simulink model "SimulatorModel"  (Simulink 10.1)
settings: Solver=ode8  StartTime=0.0  StopTime=100000  FixedStep=time_step  RelTol=1e-3
StartFcn:
  | copyfile(char(CurrentFolder + "\3DModels\" + string(MODELO_3D)), char(CurrentFolder + "\" + string(MODELO_3D)));
StopFcn:
  | delete(MODELO_3D)
values from neighbouring files (symbols this model uses):
  Aileron_Trim = 0    [InitialState.m]
  Elevator_Trim = 0    [InitialState.m]    (also in main.m)
  Engine_Trim = 0    [InitialState.m]    (also in main.m)
  GeoDate_Ap = GeoDate_ApIndex(randi([1,length(GeoDate_ApIndex)],1))    [main.m]
  GeoDate_Day = datenum(char(today("datetime")),'dd-mmm-yyyy')-datenum(char("01-January-" + GeoDate_Clock(1)'),'dd-mmm-yyyy')    [main.m]
  GeoDate_LatLongElv = [dms2degrees(Lat) dms2degrees(Long) Elv]    [main.m]
  GeoDate_Time = GeoDate_Clock(4) * 3600 + GeoDate_Clock(5) * 60 + GeoDate_Clock(6)    [main.m]
  Mission = 0    [main.m]
  Mission_Data = [0,0,0,0,0;0,0,0,0,0;0,0,0,0,0]    [main.m]
  p_ini = 0    [InitialState.m]
  phi_ini = 0*pi/180    (= 0)    [InitialState.m]    (also in main.m)
  psi_ini = 0*pi/180    (= 0)    [InitialState.m]    (also in main.m = -1.1815879036)
  q_ini = 0    [InitialState.m]
  r_ini = 0    [InitialState.m]
  Rudder_Trim = 0    [InitialState.m]
  theta_ini = 1*pi/180    (= 0.0174532925199)    [InitialState.m]    (also in main.m = 0)
  time_step = 0.200    (= 0.2)    [main.m]
  u_ini = 0    [InitialState.m]    (also in main.m)
  v_ini = 0    [InitialState.m]    (also in main.m)
  w_ini = 0    [InitialState.m]    (also in main.m)
  x_ini = 0    [InitialState.m]    (also in main.m)
  y_ini = 0    [InitialState.m]    (also in main.m)
  z_ini = h    (= 7350)    [InitialState.m]    (also in main.m = 0)
undefined symbols (not defined in the file or in its folder): AoA_alpha_max, AoA_beta_max, b, c, cargo_mass, CD0_interp, CD_ajus_coef, CD_beta_interp, CD_mach_reg, CDde, CDflap, CDgear, CDi, CDsb, CDsp, CL_ajus_coef, CL_alpha_interp, CL_alpha_reg, Clb, Clda_interp, CLde, Cldr, Clp, Clr, Cm0, Cm_alpha, Cmadot, Cmde_ajus_coef, Cmde_interp, Cmq, Cnb, Cndr, Cnr, Coef_Aileron_Beta, Coef_Aileron_Phi, Coef_Aileron_Rudder, Coef_Elevator_Alpha, Coef_Rudder_Aileron, Coef_Rudder_Beta, CYb, dCLflap, dfuel, dfuel0, e0_0, e1_0, e2_0, e3_0, fuel, fuel_density, fuel_max, g, Ixx, Ixz, Iyy, Izz, kCDge_interp, kCLge_interp, kCLsb, kCLsp, KT ... (+20)
libraries: aerolibconvert2 x17, aerolibutil x14, dsppolyfun x7, aerolibactuator x5, sharedtransform x4, robotcorelib x4, simulink x3, aerolibanim x3, visionstatistics x3, vrlib x2, dspsnks4 x1, dspvision x1
(part 1 of 3)
settings Model: Creator=AngelDanielVR_2022  LastModifiedBy=eldan  EnablePacing=on
settings Model: SuppressorTable=|
  | <?xml version="1.0" encoding="UTF-8" standalone="yes" ?>
  | <!DOCTYPE boost_serialization>
  | <boost_serialization signature="serialization::archive" version="17">
  | <DiagnosticSuppressor class_id="0" tracking_level="0" version="6">
  | 	<Table class_id="1" tracking_level="0" version="0">
  | 		<count>1</count>
  | 		<bucket_count>8</bucket_count>
  | 		<item_version>0</item_version>
  | 		<item class_id="2" tracking_level="0" version="0">
  | 			<first class_id="3" tracking_level="0" version="6">
  | 				<Source class_id="4" tracking_level="0" version="0">
  | 					<count>1</count>
  | 					<item_version>0</item_version>
  | 					<item>SimulatorModel/Fuerzas Aerodinamicas/Divide</item>
  | 				</Source>
  | 			</first>
  | 			<second class_id="5" tracking_level="0" version="6">
  | 				<SuppressedData class_id="6" tracking_level="0" version="0">
  | 					<count>1</count>
  | 					<bucket_count>8</bucket_count>
  | 					<item_version>0</item_version>
  | 					<item class_id="7" tracking_level="0" version="0">
  | 						<first class_id="8" tracking_level="0" version="6">
  | 							<ID>Simulink:blocks:DivideByZero</ID>
  | 							<Cause>
  | 								<Source>
  | 									<count>0</count>
  | 									<item_version>0</item_version>
  | 								</Source>
  | 							</Cause>
  | 						</first>
  | 						<second class_id="9" tracking_level="0" version="6">
  | 							<Comment></Comment>
  | 							<User>eldan</User>
  | 							<LastModified class_id="10" tracking_level="0" version="0">
  | 								<ptime_date class_id="11" tracking_level="0" version="0">
  | 									<date>20220312</date>
  | 								</ptime_date>
  | 								<ptime_time_duration class_id="12" tracking_level="0" version="1">
  | 									<is_special>0</is_special>
  | 									<time_duration_hours>20</time_duration_hours>
  | 									<time_duration_minutes>16</time_duration_minutes>
  | 									<time_duration_seconds>47</time_duration_seconds>
  | 									<time_duration_fractional_seconds>0</time_duration_fractional_seconds>
  | 								</ptime_time_duration>
  | 							</LastModified>
  | 							<SuppressionType>0</SuppressionType>
  | 						</second>
  | 					</item>
  | 				</SuppressedData>
  | 			</second>
  | 		</item>
  | 	</Table>
  | </DiagnosticSuppressor>
  | 
  | </boost_serialization>
  | 
  | </boost_serialization>
settings DataIOCC: SaveFormat=Dataset  ReturnWorkspaceOutputs=on  ReturnWorkspaceOutputsName=Simulation
settings OptimizationCC: LifeSpan=auto
settings DebuggingCC: UnderspecifiedInitializationDetection=Simplified  MergeDetectMultiDrivingBlocksExec=error  SFUnexpectedBacktrackingDiag=error  SFNoUnconditionalDefaultTransitionDiag=error  SFExecutionAtInitializationDiag=warning  ArithmeticOperatorsInVariantConditions=error
settings HardwareCC: ProdBitPerPointer=64  ProdBitPerSizeT=64  ProdBitPerPtrDiffT=64  ProdLargestAtomicFloat=Float  ProdIntDivRoundTo=Zero  ProdEndianess=LittleEndian  ProdWordSize=64  ProdHWDeviceType=Intel->x86-64 (Windows64)
settings ModelReferenceCC: PropagateSignalLabelsOutOfModel=on
settings SFSimCC: SimUseLocalCustomCode=on  CustomCodeUndefinedFunction=FilterOut
settings RTWCC: RTWUseLocalCustomCode=on
settings CodeAppCC: StateflowObjectComments=off
settings GRTTargetCC: TargetLangStandard=C99 (ISO)  CombineOutputUpdateFcns=on  GRTInterface=off
settings ConfigComp: CovMetricSettings=dwe  CovHtmlReporting=off  CovSaveCumulativeToWorkspaceVar=off  CovSaveSingleToWorkspaceVar=off  CovExternalEMLEnable=on

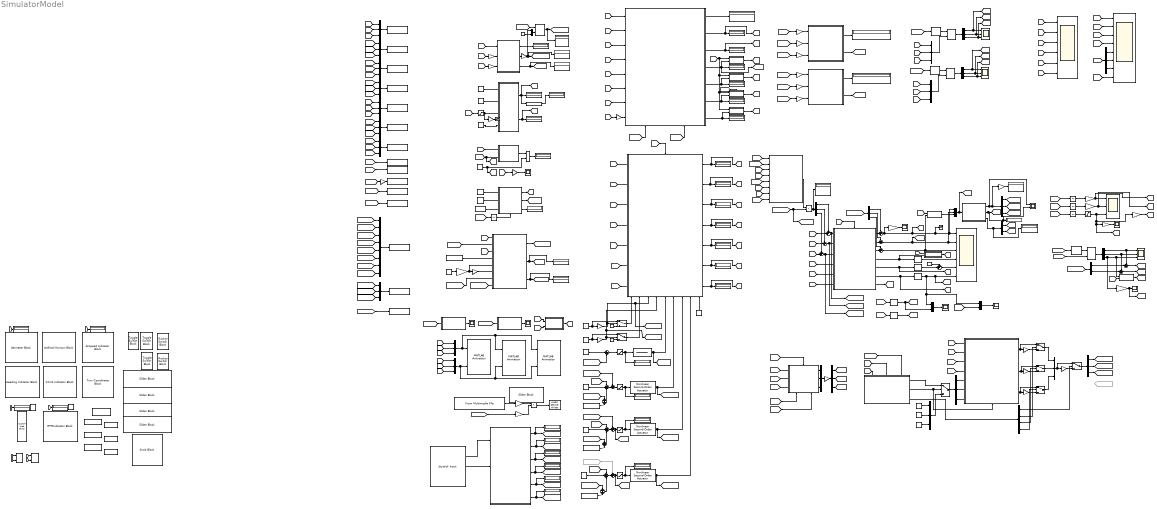
== system SimulatorModel ==
  note: Engine %
  note: Fuel %
  note: Auto-Pilot
  note: ft
  note: ALT
  note: knots
  note: VEL
  note: deg
  note: HDG
  note: Wind Control
  note: Flight Assistance
  note: Gear
  note: Speedbrakes
  note: Spoilers
  "       " : Constant  Value=mass0
  "          " : Constant  Value=fuel
  "               " : Constant  Value=cargo_mass
  6DOF (Ejes Cuerpo) : Subsystem
      settings: PortSchema="{\"entries\":[{\"content\":{\"sides\":[{\"content\":{\"connectorIds\":[\"In1\",\"In2\",\"In3\",\"In4\",\"In5\",\"In6\"]},\"type\":\"ConnectorPlacement.EquallySpacedRectSide\",\"uuid\":\"e513d8e1-8e1d-4192-a11f-b667e9f47cd4\"},{\"content\":{\"connectorIds\":[\"Out1\",\"Out2\",\"Out3\",\"Out4\",\"Out5\",\"Out6\",\"Out7\"],\"side\":\"RIGHT\"},\"type\":\"ConnectorPlacement.EquallySpacedRectSide\",\"uuid\":\"fc5bffb2-c734-419d-b044-938a48a874f8\"},{\"content\":{\"connectorIds\":[\"In7\"],\"side\":\"TOP\"},\"type\":\"ConnectorPlacement.EquallySpacedRectSide\",\"uuid\":\"e4739993-ca2d-4725-a873-646bc3002720\"}]},\"type\":\"ConnectorPlacement.EquallySpacedConnector\",\"uuid\":\"4b4d31a3-c546-405e-8f8c-e6c94c8ecc35\"}],\"packageUris\":[\"http://schema.mathworks.com/mf0/Connector/19700101\"],\"version\":\"1.0\"}"
  ALT : Gain
  Abs : Abs
  Aileron Position : Constant  Value=0
  Airspeed Indicator1 : AirspeedIndicatorBlock  LabelPosition=Hide  ScaleMin=60  ScaleMax=717  ScaleColors=DataTag1
  Altimeter : AltimeterBlock  LabelPosition=Hide
  Altitude Navigation : simulink/Sinks/XY Graph  xmin=0  xmax=500  ymin=0  ymax=8000  st=1
  Altura Autopiloto : Constant  Value=24114
  Angle Conversion{,1..2,6..7} (5 alike) : aerolibconvert2/Angle Conversion  IU=rad  OU=deg
  Animacion Aeronave 3D Back : aerolibanim/MATLAB Animation  Tag=Matlab Animation 6 DOF  Vehicles=1  Geometries=MODELO_3D  BoundingBoxCoordinates=MODELO_3D_Data_Box  CameraOffset=MODELO_3D_DataBack_Offset  CameraViewAngle=2  SampleTime=time_step  FigurePosition=[37,8.020000e+01,396,3.184000e+02]
      settings: SourceProductBaseCode=AE
  Animacion Aeronave 3D ISO : aerolibanim/MATLAB Animation  Tag=Matlab Animation 6 DOF  Vehicles=1  Geometries=MODELO_3D  BoundingBoxCoordinates=MODELO_3D_Data_Box  CameraOffset=MODELO_3D_DataISO_Offset  CameraViewAngle=2  SampleTime=time_step  FigurePosition=[1.018000e+02,4.602000e+02,4.008000e+02,3.080000e+02]
      settings: SourceProductBaseCode=AE
  Animacion Aeronave 3D Side : aerolibanim/MATLAB Animation  Tag=Matlab Animation 6 DOF  Vehicles=1  Geometries=MODELO_3D  BoundingBoxCoordinates=MODELO_3D_Data_Box  CameraOffset=MODELO_3D_DataSide_Offset  CameraViewAngle=2  SampleTime=time_step  FigurePosition=[7.138000e+02,1.226000e+02,7.064000e+02,4.224000e+02]
      settings: SourceProductBaseCode=AE
  Artificial Horizon : ArtificialHorizonBlock  LabelPosition=Hide
  Asistencia en Vuelo : Subsystem
      settings: PortSchema="{\"entries\":[{\"content\":{\"sides\":[{\"content\":{\"connectorIds\":[\"In1\",\"In2\",\"In3\"]},\"type\":\"ConnectorPlacement.EquallySpacedRectSide\",\"uuid\":\"2b982a28-1fea-4abf-9de3-2f9de9411225\"},{\"content\":{\"connectorIds\":[\"Out1\",\"Out2\",\"Out3\"],\"side\":\"RIGHT\"},\"type\":\"ConnectorPlacement.EquallySpacedRectSide\",\"uuid\":\"2f2ccd38-6861-4845-9efc-cf53ec30643e\"},{\"content\":{\"connectorIds\":[\"In4\"],\"side\":\"TOP\"},\"type\":\"ConnectorPlacement.EquallySpacedRectSide\",\"uuid\":\"10eced36-af19-42c5-8d6d-546cf7986fc2\"},{\"content\":{\"connectorIds\":[\"In5\",\"In6\"],\"side\":\"BOTTOM\"},\"type\":\"ConnectorPlacement.EquallySpacedRectSide\",\"uuid\":\"486c9866-702d-4628-bb5b-4c00364c2671\"}]},\"type\":\"ConnectorPlacement.EquallySpacedConnector\",\"uuid\":\"8a4f78da-55c7-44fd-bc59-53ea1e78315a\"}],\"packageUris\":[\"http://schema.mathworks.com/mf0/Connector/19700101\"],\"version\":\"1.0\"}"
  Audio Device Writer : dspsnks4/Audio Device Writer  Driver=DirectSound  Device=Default  InheritSampleRate=on  SampleRate=44100  BitDepth=16-bit integer  BufferSize=4096  NumBuffers=10  DefaultOutputChannelMapping=on  OutputChannelMapping=1:2  OutputNumUnderrunSamples=off  DriverIdx=1  DeviceWarnFlag=''
  Auto-Piloto : Subsystem
      settings: PortSchema="{\"entries\":[{\"content\":{\"sides\":[{\"content\":{\"connectorIds\":[\"In1\",\"In2\",\"In3\",\"In4\",\"In5\",\"In6\",\"In7\"]},\"type\":\"ConnectorPlacement.EquallySpacedRectSide\",\"uuid\":\"540fb58f-a9c8-4ad4-9356-3d566afe9f2d\"},{\"content\":{\"connectorIds\":[\"Out1\",\"Out2\",\"Out3\"],\"side\":\"RIGHT\"},\"type\":\"ConnectorPlacement.EquallySpacedRectSide\",\"uuid\":\"002c5e45-ef8b-4bc5-a5df-6a486272560c\"},{\"content\":{\"connectorIds\":[],\"side\":\"TOP\"},\"type\":\"ConnectorPlacement.EquallySpacedRectSide\",\"uuid\":\"228a911a-da3e-4d63-8be4-0617bff602d3\"},{\"content\":{\"connectorIds\":[\"In8\"],\"side\":\"BOTTOM\"},\"type\":\"ConnectorPlacement.EquallySpacedRectSide\",\"uuid\":\"7f0ae31e-3482-443b-902a-85f32887179f\"}]},\"type\":\"ConnectorPlacement.EquallySpacedConnector\",\"uuid\":\"3a82b01a-db7e-44ad-a37b-33b4a4c7be3f\"}],\"packageUris\":[\"http://schema.mathworks.com/mf0/Connector/19700101\"],\"version\":\"1.0\"}"
  Brake Force System : Subsystem
  Climb Rate Indicator : ClimbIndicatorBlock  LabelPosition=Hide  ScaleMax=20000
  Constant : Constant  Value=Aileron_Trim
  Constant1 : Constant  Value=Rudder_Trim
  Constant2 : Constant  Value=Elevator_Trim
  Constant3 : Constant  Value=Engine_Trim
  Constant4 : Constant
  Constant5 : Constant
  Constant6 : Constant  Value=0
  Constant7 : Constant  Value=90
  Control ON/OFF Asistencia en Vuelo : Gain
  Demux{,1..3,5..8,10..11} (10 alike) : Demux  Outputs=3
  Demux12 : Demux
  Demux4 : Demux  Outputs=2
  Demux9 : Demux  Outputs=2
  Densidad : Display
  Densidad a  Nivel del Mar : Constant  Value=rho0
  Dirección Autopiloto : Constant  Value=22
  Display{,1..12} (13 alike) : Display
  Edit : EditField  LabelPosition=Hide  ShowInitialText=on  Alignment=Center
  Edit1 : EditField  LabelPosition=Hide  ShowInitialText=on  Alignment=Center
  Edit2 : EditField  LabelPosition=Hide  ShowInitialText=on  Alignment=Center
  Ejes Cuerpo : Scope  NumInputPorts=6
  Ejes Globales : Scope  NumInputPorts=3
  Ejes Globales3 : Scope  NumInputPorts=3
  Elevator Position : Constant  Value=0
  Engine % : Display
  "Engine %  " : Display
  Engine Alert : Subsystem
  Flaps Position : Constant  Value=0
  From Multimedia File : dspvision/From Multimedia File  inputFilename=SOUND_EFECT1  readRange=[1 Inf]  loop=on  numPlays=inf  outputStreams=Audio only  videoDataType=single  audioDataType=double  inheritSampleTime=off  userDefinedSampleTime=time_step  noAudioOutput=off  isIntensityVideo=off  fourcc=RGB  colorVideoFormat=Separate color signals  outputEOF=off  dataOrg=Column-major  audioFrameSize=1024  computeAudioFrameSize=off  outSamplingMode=Sample based
  From153 : From  Commented=on  GotoTag=Aileron_AutoPilot
  Fuel % : Display
  Fuel %1 : Display
  Fuel %2 : Display
  Fuel Alert : Subsystem
  Fuel Flow : Display
      settings: Decimation=2
  Fuerza Lateral : Display
  Fuerzas Aerodinamicas : Subsystem
      settings: PortSchema="{\"entries\":[{\"content\":{\"sides\":[{\"content\":{\"connectorIds\":[\"In1\",\"In2\",\"In3\",\"In4\",\"In5\",\"In6\",\"In7\"]},\"type\":\"ConnectorPlacement.EquallySpacedRectSide\",\"uuid\":\"3250c387-4f55-4b28-834f-fee09e54f43c\"},{\"content\":{\"connectorIds\":[\"Out1\",\"Out2\",\"Out3\",\"Out4\",\"Out5\",\"Out6\",\"Out7\"],\"side\":\"RIGHT\"},\"type\":\"ConnectorPlacement.EquallySpacedRectSide\",\"uuid\":\"40541228-441d-4bb0-b352-01b290a375ec\"},{\"content\":{\"connectorIds\":[\"In8\"],\"side\":\"TOP\"},\"type\":\"ConnectorPlacement.EquallySpacedRectSide\",\"uuid\":\"ce027dbc-72c9-4eaa-8f9d-4a9b52d929e1\"},{\"content\":{\"connectorIds\":[\"In9\",\"In10\",\"In11\",\"In12\",\"In13\",\"In14\",\"In15\",\"In16\",\"In17\"],\"side\":\"BOTTOM\"},\"type\":\"ConnectorPlacement.EquallySpacedRectSide\",\"uuid\":\"4afb7921-1bd6-40c2-a379-9d150abe5192\"}]},\"type\":\"ConnectorPlacement.EquallySpacedConnector\",\"uuid\":\"bf5ac778-d8f5-40f6-900f-aa06f3ea431b\"}],\"packageUris\":[\"http://schema.mathworks.com/mf0/Connector/19700101\"],\"version\":\"1.0\"}"
  Fuerzas Ejes Cuerpo1 : Display
  Fx_c : Display
  Fy_c : Display
  Fz_c : Display
  Gain{1,10..15} (7 alike) : Gain  Gain=-1
  Gain2 : Gain  Gain=-g
  Gain24 : Gain  Gain=1/100
  Gain25 : Gain
  Gain3 : Gain  Gain=1/1000
  Gain4 : Gain  Gain=1/1000
  Gain5 : Gain  Gain=fuel_max
  Gain6 : Gain  Gain=1/1000
  Gain7 : Gain  Gain=1.94
  Gain8 : Gain  Gain=1000
  Gain9 : Gain  Gain=1000
  Gear Position : Constant  Value=0
  Giro de Fuerzas a Ejes Cuerpo QUATERNIONES : Subsystem
      settings: PortSchema="{\"entries\":[{\"content\":{\"sides\":[{\"content\":{\"connectorIds\":[\"In1\",\"In2\",\"In3\",\"In4\",\"In5\",\"In6\",\"In7\",\"In8\"]},\"type\":\"ConnectorPlacement.EquallySpacedRectSide\",\"uuid\":\"1cdf8b7c-a170-4eac-a859-8c0a1fcd9a61\"},{\"content\":{\"connectorIds\":[\"Out1\",\"Out2\",\"Out3\",\"Out4\",\"Out5\",\"Out6\",\"Out7\"],\"side\":\"RIGHT\"},\"type\":\"ConnectorPlacement.EquallySpacedRectSide\",\"uuid\":\"8933edc5-ca20-448c-9ac2-7633dd75b8dc\"},{\"content\":{\"connectorIds\":[],\"side\":\"TOP\"},\"type\":\"ConnectorPlacement.EquallySpacedRectSide\",\"uuid\":\"457e456d-9a46-43dd-ad19-0337464f22e7\"},{\"content\":{\"connectorIds\":[\"In9\",\"In10\"],\"side\":\"BOTTOM\"},\"type\":\"ConnectorPlacement.EquallySpacedRectSide\",\"uuid\":\"55b3d68e-8e66-45f1-9454-3489a38eee0c\"}]},\"type\":\"ConnectorPlacement.EquallySpacedConnector\",\"uuid\":\"3b4d2913-db28-4058-985d-03cab48c44be\"}],\"packageUris\":[\"http://schema.mathworks.com/mf0/Connector/19700101\"],\"version\":\"1.0\"}"
  Goto5 : Goto  Commented=on  GotoTag=Aileron_AutoPilot
  Gravedad : Constant  Value=g
  HDG : Gain  Gain=0
  Heading Indicator : HeadingIndicatorBlock  LabelPosition=Hide
  Incidence Angles : Display
  Integrator1 : Integrator  InitialCondition=y_ini
  Integrator2 : Integrator  InitialCondition=x_ini
  Integrator3 : Integrator  InitialCondition=z_ini
  Joystick Input : vrlib/Joystick Input  joyid=1  adjustports=on  forcefeed=off
  Knob : KnobBlock  ScaleMax=1
  Lamp : LampBlock  LabelPosition=Hide  DefaultColor=DataTag16  States=DataTag17
  Lamp1 : LampBlock  LabelPosition=Hide  DefaultColor=DataTag19  States=DataTag20
  Mach : Display
  Master : Gain  Gain=0
  Matriz de Cambio de Ejes Globales a Cuerpo QUATERNIONES : Subsystem
  Matriz de Cambio de Ejes Viento a Cuerpo QUATERNIONES : Subsystem
  Matriz de Giro : Display
  Matriz de Giro1 : Display
  Modelo Atmosfera ISA : Subsystem
  Momento de Alabeo : Display
  Momento de Cabeceo : Display
  Momento de Guiñada : Display
  Monitor General : Scope  NumInputPorts=8
  Monitor de Fuerzas Ejes Cuerpo : Scope  NumInputPorts=6
  Monitor de Fuerzas Ejes Globales : Scope  NumInputPorts=3
  Monitor de Momentos Ejes Globales1 : Scope  NumInputPorts=3
  Mux{,1,3..6,8,10..18} (16 alike) : Mux  Inputs=3
  Mux19 : Mux  Inputs=2
  Mux2 : Mux  Inputs=2
  Mux7 : Mux  Inputs=2
  Mux9 : Mux  Inputs=8
  Mx_c : Display
  My_c : Display
  Mz_c : Display
  Nonlinear Second-Order Actuator : aerolibactuator/Nonlinear Second-Order Actuator  wn_fin=4  z_fin=1  fin_max=90*pi/180  fin_min=-90*pi/180  fin_maxrate=500*pi/180/1.9/2  fin_act_0=Elevator_Trim  fin_act_vel=0
      settings: SourceProductBaseCode=AE
  Nonlinear Second-Order Actuator1 : aerolibactuator/Nonlinear Second-Order Actuator  wn_fin=4  z_fin=1  fin_max=90*pi/180  fin_min=-90*pi/180  fin_maxrate=500*pi/180/1.9/2  fin_act_0=Rudder_Trim  fin_act_vel=0
      settings: SourceProductBaseCode=AE
  Nonlinear Second-Order Actuator2 : aerolibactuator/Nonlinear Second-Order Actuator  wn_fin=4  z_fin=1  fin_max=90*pi/180  fin_min=-90*pi/180  fin_maxrate=500*pi/180/1.9/2  fin_act_0=Aileron_Trim  fin_act_vel=0
      settings: SourceProductBaseCode=AE
  Normal1 : Subsystem
  Numero de Motores : Gain  Gain=NMotores
  ON/OFF Spoiler : Gain  Gain=0
  ON/OFF  SpeedBrake : Gain  Gain=0
  Porcentaje de Motor : Gain  Gain=0
  Product1 : Product
  Product3 : Product
  Product4 : Product
  Quaternion Inverse : aerolibutil/Quaternion Inverse
  Quaternion Inverse1 : aerolibutil/Quaternion Inverse
  Quaternion Inverse2 : aerolibutil/Quaternion Inverse
  Quaternion Rotation{1..3,6} (4 alike) : aerolibutil/Quaternion Rotation
  RPM Indicator : RPMIndicatorBlock  LabelPosition=Hide  ScaleColors=DataTag22
  Resistencia : Display
  Rocker Switch : RockerSwitchBlock  LabelPosition=Hide  Values=DataTag24
  Rocker Switch1 : RockerSwitchBlock  LabelPosition=Hide  Values=DataTag26
  Rudder Position : Constant  Value=0
  Saturation : Saturate  UpperLimit=1  LowerLimit=-1
  Saturation1 : Saturate  UpperLimit=1  LowerLimit=-1
  Saturation2 : Saturate  UpperLimit=1  LowerLimit=-1
  Saturation3 : Saturate  UpperLimit=OperativeCeiling  LowerLimit=0
  Saturation7 : Saturate  UpperLimit=inf  LowerLimit=0
  Saturation8 : Saturate  UpperLimit=1  LowerLimit=0
  Scope{,4..5,7..8,13..15} (8 alike) : Scope
  Scope6 : Scope  NumInputPorts=2
  Slider : SliderBlock  ScaleMax=1  TickInterval=0.125
  Slider Switch : SliderSwitchBlock  LabelPosition=Hide  Values=DataTag29
  Slider Switch1 : SliderSwitchBlock  LabelPosition=Hide  Values=DataTag31
  Slider Switch2 : SliderSwitchBlock  LabelPosition=Hide  Values=DataTag33
  Slider Switch3 : SliderSwitchBlock  LabelPosition=Hide  Values=DataTag35
  Slider1 : SliderBlock  ScaleMin=-1  ScaleMax=1  TickInterval=0.25
  Slider2 : SliderBlock  ScaleMin=-1  ScaleMax=1  TickInterval=0.25
  Slider3 : SliderBlock  ScaleMin=-1  ScaleMax=1  TickInterval=0.25
  Slider4 : SliderBlock  LabelPosition=Hide  ScaleMax=2
  SpeedBrake : Constant  Value=kCLsb
  Spoiler : Constant  Value=kCLsp
  Subsystem q : Subsystem
  Subsystem10 : Subsystem
  Subsystem11 : Subsystem
  Subsystem12 : Subsystem
  Subsystem13 : Subsystem
      settings: PortSchema="{\"entries\":[{\"content\":{\"sides\":[{\"content\":{\"connectorIds\":[\"In1\",\"In2\"]},\"type\":\"ConnectorPlacement.EquallySpacedRectSide\",\"uuid\":\"9824aea0-cc81-4e51-b2d2-cbf2e465da36\"},{\"content\":{\"connectorIds\":[\"Out1\"],\"side\":\"RIGHT\"},\"type\":\"ConnectorPlacement.EquallySpacedRectSide\",\"uuid\":\"ba6234b1-8308-4857-b5c2-42009c2616e8\"},{\"content\":{\"connectorIds\":[\"In3\"],\"side\":\"TOP\"},\"type\":\"ConnectorPlacement.EquallySpacedRectSide\",\"uuid\":\"2071bb01-be77-48a3-b753-3d3e0f95e4a1\"}]},\"type\":\"ConnectorPlacement.EquallySpacedConnector\",\"uuid\":\"c53ca202-57e3-4806-b8f0-972dff98310e\"}],\"packageUris\":[\"http://schema.mathworks.com/mf0/Connector/19700101\"],\"version\":\"1.0\"}"
  Subsystem14 : Subsystem
  Subsystem15 : Subsystem
      settings: PortSchema="{\"entries\":[{\"content\":{\"sides\":[{\"content\":{\"connectorIds\":[]},\"type\":\"ConnectorPlacement.EquallySpacedRectSide\",\"uuid\":\"c504bf1c-e23e-41e1-ae5f-6f3bb65b3b4c\"},{\"content\":{\"connectorIds\":[\"Out1\",\"Out2\",\"Out3\"],\"side\":\"RIGHT\"},\"type\":\"ConnectorPlacement.EquallySpacedRectSide\",\"uuid\":\"32c4c404-12e9-43f3-8b9d-576d77bea652\"},{\"content\":{\"connectorIds\":[\"In1\",\"In2\",\"In3\"],\"side\":\"TOP\"},\"type\":\"ConnectorPlacement.EquallySpacedRectSide\",\"uuid\":\"b1fde21f-409d-4890-9c14-ccab09f359fc\"}]},\"type\":\"ConnectorPlacement.EquallySpacedConnector\",\"uuid\":\"dc4b4957-b4fd-4424-a8a9-3d4e41803d55\"}],\"packageUris\":[\"http://schema.mathworks.com/mf0/Connector/19700101\"],\"version\":\"1.0\"}"
  Subsystem16 : Subsystem
  Subsystem17 : Subsystem
  Subsystem2 : Subsystem
  Subsystem3 : Subsystem
  Subsystem4 : Subsystem
  Subsystem6 : Subsystem
  Subsystem9 : Subsystem
      settings: PortSchema="{\"entries\":[{\"content\":{\"sides\":[{\"content\":{\"connectorIds\":[\"In1\",\"In2\",\"In3\"]},\"type\":\"ConnectorPlacement.EquallySpacedRectSide\",\"uuid\":\"00044d68-f698-4012-ab03-09b54e6a53f3\"},{\"content\":{\"connectorIds\":[\"Out1\",\"Out2\",\"Out3\"],\"side\":\"RIGHT\"},\"type\":\"ConnectorPlacement.EquallySpacedRectSide\",\"uuid\":\"4a64a270-e9d8-4555-85a1-9bbba4f5cfb3\"},{\"content\":{\"connectorIds\":[],\"side\":\"TOP\"},\"type\":\"ConnectorPlacement.EquallySpacedRectSide\",\"uuid\":\"494e8594-af25-482d-897a-db0a5de199af\"},{\"content\":{\"connectorIds\":[\"In4\"],\"side\":\"BOTTOM\"},\"type\":\"ConnectorPlacement.EquallySpacedRectSide\",\"uuid\":\"fbd05360-1415-4579-a7a9-b7a753fb6aac\"}]},\"type\":\"ConnectorPlacement.EquallySpacedConnector\",\"uuid\":\"5553b20b-1ba8-42cc-9c0c-112a49b3f965\"}],\"packageUris\":[\"http://schema.mathworks.com/mf0/Connector/19700101\"],\"version\":\"1.0\"}"
  Sum : Sum  Inputs=-++
  Sum1 : Sum  Inputs=-++
  Sum{10..12,14..17,19..20} (9 alike) : Sum  Inputs=++|
  Sum13 : Sum  Inputs=|++
  Sum2 : Sum  Inputs=-++
  Sum3 : Sum
  Sum4 : Sum
  Sum5 : Sum
  Sum7 : Sum  Inputs=-+|
  Sum8 : Sum  Inputs=-+|
  Sum9 : Sum  Inputs=-+|
  Superficie Alar : Constant  Value=S
  Sustentacion : Display
  Switch{1..2,4..8} (7 alike) : Switch  Criteria=u2 ~= 0
  Temperatura : Display
      settings: Decimation=2
  Temperatura a  Nivel del Mar : Constant  Value=temp0
  Temperatura1 : Display
      settings: Decimation=2
  Temperature Conversion : aerolibconvert2/Temperature Conversion  IU=K  OU=C
      settings: SourceProductBaseCode=AE
  Terminator1 : Terminator
  Terminator3 : Terminator
  To Workspace : ToWorkspace  VariableName=Position  SampleTime=-1
      settings: Save2DSignal=2-D array (concatenate along first dimension)
  To Workspace1 : ToWorkspace  VariableName=Global_Velocity  SampleTime=-1
      settings: Save2DSignal=2-D array (concatenate along first dimension)
  To Workspace10 : ToWorkspace  VariableName=Distance  SampleTime=-1
      settings: Save2DSignal=2-D array (concatenate along first dimension)
  To Workspace11 : ToWorkspace  VariableName=Body_Forces  SampleTime=-1
      settings: Save2DSignal=2-D array (concatenate along first dimension)
  To Workspace12 : ToWorkspace  VariableName=Actuators  SampleTime=-1
      settings: Save2DSignal=2-D array (concatenate along first dimension)
  To Workspace13 : ToWorkspace  VariableName=Body_Velocity  SampleTime=-1
      settings: Save2DSignal=2-D array (concatenate along first dimension)
  To Workspace14 : ToWorkspace  VariableName=Global_Forces  SampleTime=-1
      settings: Save2DSignal=2-D array (concatenate along first dimension)
  To Workspace2 : ToWorkspace  VariableName=Global_Moments  SampleTime=-1
      settings: Save2DSignal=2-D array (concatenate along first dimension)
  To Workspace3 : ToWorkspace  VariableName=Global_Angles  SampleTime=-1
      settings: Save2DSignal=2-D array (concatenate along first dimension)
  To Workspace4 : ToWorkspace  VariableName=Wind_Angles  SampleTime=-1
      settings: Save2DSignal=2-D array (concatenate along first dimension)
  To Workspace5 : ToWorkspace  VariableName=Alpha  SampleTime=-1
      settings: Save2DSignal=2-D array (concatenate along first dimension)
  To Workspace6 : ToWorkspace  VariableName=Beta  SampleTime=-1
      settings: Save2DSignal=2-D array (concatenate along first dimension)
  To Workspace7 : ToWorkspace  VariableName=Body_Moments  SampleTime=-1
      settings: Save2DSignal=2-D array (concatenate along first dimension)
  To Workspace8 : ToWorkspace  VariableName=Fuel  SampleTime=-1
      settings: Save2DSignal=2-D array (concatenate along first dimension)
  To Workspace9 : ToWorkspace  VariableName=Lat_Lon  SampleTime=-1
      settings: Save2DSignal=2-D array (concatenate along first dimension)
  Toggle Switch : ToggleSwitchBlock  LabelPosition=Hide  Values=DataTag42
  Toggle Switch1 : ToggleSwitchBlock  LabelPosition=Hide  Values=DataTag44
  Toggle Switch2 : ToggleSwitchBlock  LabelPosition=Hide  Values=DataTag46
  Traccion : Display
  Traccion por Motor : Constant  Value=T
  Transfer Fcn1 : TransferFcn  Denominator=[2 4 1]
  Turn Coordinator : TurnCoordinatorBlock  LabelPosition=Hide
  VEL : Gain
  Velocidad Autopiloto : Constant  Value=300
  Vertical Gauge : CustomWebBlock  LabelPosition=Hide  ShowInitialText=on  Configuration="{\"components\":[{\"name\":\"LinearScaleComponent\",\"settings\":{\"bounds\":{\"max\":100,\"min\":0,\"tickInterval\":25},\"labelColor\":[250,245,199],\"labelFont\":{\"font\":\"Arial\",\"fontSize\":12},\"labelTransparency\":1,\"needleImage\":{\"size\":[21,75],\"src\":\"data:image\\/svg+xml;base64,PHN2ZyB4bWxucz0iaHR0cDovL3d3dy53My5vcmcvMjAwMC9zdmciIHhtbG5zOnhsaW5rPSJodHRwOi8vd3d3LnczLm9yZy8xOTk5L3hsaW5rIiB2aWV3Qm94PSIwIDAgMjEgNzUiPjxkZWZzPjxzdHlsZT4uY2xzLTF7ZmlsbDpub25lO30uY2xzLTJ7aXNvbGF0aW9uOmlzb2xhdGU7fS5jbHMtM3tjbGlwLXBhdGg6dXJsKCNjbGlwLXBhdGgpO30uY2xzLTR7b3BhY2l0eTowLjM7bWl4LWJsZW5kLW1vZGU6bXVsdGlwbHk7fS5jbHMtNXtmaWxsOiNlYjI2Mjk7fTwvc3R5bGU+PGNsaXBQYXRoIGlkPSJjbGlwLXBhdGgiIHRyYW5zZm9y ...(+1928 chars)\",\"srcOrientation\":\"horizontal\"},\"needleOffset\":[-0.01094391244870041,0],\"needleSize\":{\"height\":0.11960078534031414,\"width\":0.7589285714285714},\"position\":[0.015887605042016806,0.06986607142857143,0.8,0.9641544117647058],\"scaleColorSize\":0.24,\"scaleColors\":[],\"scaleColorsSize\":0.2,\"tickColor\":[250,245,200],\"tickTransparency\":1,\"valueBarColor\":[23,89,176],\"valueBarSize\":0.23,\"valueBarTransparency\":1}},{\"name\":\"BackgroundImageComponent\",\"settings\":{\"image\":{\"size\":[380,101],\"src\":\"data:image\\/svg+xml;base64,PHN2ZyB4bWxucz0iaHR0cDovL3d3dy53My5vcmcvMjAwMC9zdmciIHhtbG5zOnhsaW5rPSJodHRwOi8vd3d3LnczLm9yZy8xOTk5L3hsaW5rIiB2aWV3Qm94PSIwIDAgMzgwIDEwMSI+PGRlZnM+PHN0eWxlPi5jbHMtMXtmaWxsOnVybCgjbGluZWFyLWdyYWRpZW50KTt9LmNscy0ye2ZpbGw6dXJsKCNsaW5lYXItZ3JhZGllbnQtMik7fS5jbHMtM3tmaWxsOnVybCgjbGluZWFyLWdyYWRpZW50LTMpO308L3N0eWxlPjxsaW5lYXJHcmFkaWVudCBpZD0ibGluZWFyLWdyYWRpZW50IiB5MT0iNTAuNSIgeDI9IjM5OS4yOCIgeTI9IjUw ...(+2216 chars)\",\"srcOrientation\":\"horizontal\"},\"position\":[0,0,1,1],\"scaleMode\":\"0\"}}],\"settings\":{\"BindingType\":\"signal\",\"fixedAspectRatio\":\"on\",\"orientation\":\"vertical\"},\"type\":\"LinearGauge\"}"
  Volumen Efecto 1 : Gain  Gain=2
  Wind Direction : Display
      settings: Decimation=2
  Wind Vectors : Display
      settings: Decimation=2
  Wind Vectors1 : Display
      settings: Decimation=2
  Wind Vectors2 : Display
      settings: Decimation=2
  XY Navigation : simulink/Sinks/XY Graph  xmin=-200  xmax=200  ymin=-200  ymax=200  st=1
  m/s to knots : Gain  Gain=1.94384
  meters to feets : Gain  Gain=3.28
  meters to feets1 : Gain  Gain=3.28
  meters to feets2 : Gain  Gain=3.28*60
  q : Display
  wires:
  Gravedad/1 -> Modelo Atmosfera ISA/1(g)
  Densidad a  Nivel del Mar/1 -> Modelo Atmosfera ISA/2(" rho0")
  Temperatura a  Nivel del Mar/1 -> Modelo Atmosfera ISA/4(temp0)
  Modelo Atmosfera ISA/1(temp) -> Temperature Conversion/1, [temp], Temperatura/1
  Modelo Atmosfera ISA/2(rho) -> [rho], Densidad/1
  [rho] -> Subsystem q/1(rho)
  Superficie Alar/1 -> [S], Product1/2
  Subsystem q/1(q) -> Product1/1
  Traccion por Motor/1 -> Numero de Motores/1
  Numero de Motores/1 -> Subsystem17/5(Tracción Máxima), Porcentaje de Motor/1
  Matriz de Cambio de Ejes Viento a Cuerpo QUATERNIONES/2(Quat) -> [QuaterGiro_VC]
  Matriz de Cambio de Ejes Viento a Cuerpo QUATERNIONES/1(Matrix) -> Matriz de Giro/1
  Gain2/1 -> Giro de Fuerzas a Ejes Cuerpo QUATERNIONES/8(Peso)
  [L] -> Giro de Fuerzas a Ejes Cuerpo QUATERNIONES/1(Lift)
  Giro de Fuerzas a Ejes Cuerpo QUATERNIONES/1("[F,M]") -> Fuerzas Ejes Cuerpo1/1
  [My] -> Giro de Fuerzas a Ejes Cuerpo QUATERNIONES/5(My)
  [mass] -> Gain2/1
  [D] -> Giro de Fuerzas a Ejes Cuerpo QUATERNIONES/2(Drag)
  [Trac] -> Giro de Fuerzas a Ejes Cuerpo QUATERNIONES/7(Trac)
  [S] -> Fuerzas Aerodinamicas/4(S [m^2])
  [temp] -> Fuerzas Aerodinamicas/1(temp [K])
  Fuerzas Aerodinamicas/5(My) -> [My], Momento de Cabeceo/1
  Fuerzas Aerodinamicas/7(Mach) -> [Mach], Mach/1
  [rho] -> Fuerzas Aerodinamicas/2(rho [kg/m^3])
  SpeedBrake/1 -> Switch1/1, ON/OFF  SpeedBrake/1
  ON/OFF  SpeedBrake/1 -> Switch1/2, [Speedbrake_Total], Fuerzas Aerodinamicas/11(Speedbrake Pos)
  Spoiler/1 -> Switch2/1, ON/OFF Spoiler/1
  ON/OFF Spoiler/1 -> Switch2/2, Fuerzas Aerodinamicas/12(Spoiler Pos), [Spoiler_Total]
  Fuerzas Aerodinamicas/3(Yy) -> [Y], Fuerza Lateral/1
  [Y] -> Giro de Fuerzas a Ejes Cuerpo QUATERNIONES/3(SideForce)
  Fuerzas Aerodinamicas/4(Mx) -> [Mx], Momento de Alabeo/1
  [Mx] -> Giro de Fuerzas a Ejes Cuerpo QUATERNIONES/4(Mx)
  Giro de Fuerzas a Ejes Cuerpo QUATERNIONES/2(Fx_c) -> [Fx_c], Fx_c/1  "Fx"
  Giro de Fuerzas a Ejes Cuerpo QUATERNIONES/3(Fy_c) -> Fy_c/1, [Fy_c]  "Fy"
  Giro de Fuerzas a Ejes Cuerpo QUATERNIONES/4(Fz_c) -> [Fz_c_brake], Subsystem10/2(Fz), Fz_c/1  "Fz"
  [Mx_c] -> 6DOF (Ejes Cuerpo)/4(Mx Cuerpo)
  [Mz_c] -> 6DOF (Ejes Cuerpo)/6(Mz Cuerpo)
  Sum7/1 -> m/s to knots/1, [IAS], Terminator3/1, Mux/1, Ejes Cuerpo/1  "Vx"
  Sum8/1 -> [Vy_body], Ejes Cuerpo/2, Mux/2  "Vy"
  Sum9/1 -> Subsystem12/2(Vz), Ejes Cuerpo/3  "Vz"
  6DOF (Ejes Cuerpo)/4(theta) -> Subsystem14/2(theta), Angle Conversion/1
  6DOF (Ejes Cuerpo)/5(psi) -> [psi], Angle Conversion1/1  "psi"
  6DOF (Ejes Cuerpo)/6(phi) -> [phi], Angle Conversion2/1  "phi"
  Mux/1 -> Subsystem6/1(Wind Vector), [V_body]
  [psi] -> Angle Conversion7/1
  [Velocidad] -> Subsystem q/2(V), [V]
  [My_c] -> 6DOF (Ejes Cuerpo)/5(My Cuerpo)
  Angle Conversion2/1 -> Mux2/1, Mux7/1, [phi_deg], Ejes Cuerpo/6  "phi [deg]"
  Angle Conversion/1 -> Ejes Cuerpo/4  "theta [deg]"
  [QuaterGiro_GC] -> Quaternion Inverse/1
  Quaternion Inverse/1 -> Quaternion Rotation1/1
  Quaternion Rotation1/1 -> Demux/1
  Demux/3 -> Subsystem11/1(Vz), Ejes Globales/3, meters to feets2/1  "Vz"
  Demux/2 -> Sum11/1, Ejes Globales/2  "Vy"
  Demux/1 -> Sum10/1, Ejes Globales/1  "Vx"
  Demux1/1 -> [Fx_global], Monitor de Fuerzas Ejes Globales/1  "Fx"
  Demux1/2 -> [Fy_global], Monitor de Fuerzas Ejes Globales/2  "Fy"
  Quaternion Rotation2/1 -> Demux1/1
  Quaternion Inverse1/1 -> Quaternion Rotation2/1
  [QuaterGiro_GC] -> Quaternion Inverse1/1
  Demux1/3 -> [Fz_global], Monitor de Fuerzas Ejes Globales/3  "Fz"
  [theta] -> Angle Conversion6/1
  Matriz de Cambio de Ejes Globales a Cuerpo QUATERNIONES/2(Quat) -> [QuaterGiro_GC]
  Matriz de Cambio de Ejes Globales a Cuerpo QUATERNIONES/1(Matrix) -> Matriz de Giro1/1
  Integrator1/1 -> Gain4/1  "y"
  Integrator3/1 -> Saturation7/1  "z"
  Gain3/1 -> [Xpos], Ejes Globales3/1  "x [Km]"
  Integrator2/1 -> Gain3/1  "x"
  Gain4/1 -> [Ypos], Ejes Globales3/2  "y [Km]"
  Saturation7/1 -> [h], meters to feets1/1, Gain6/1, Ejes Globales3/3  "z [m]"
  Transfer Fcn1/1 -> [Flaps_Total], Fuerzas Aerodinamicas/13(Flaps Position)
  Switch2/1 -> Fuerzas Aerodinamicas/10(kCLsp)
  Switch1/1 -> Fuerzas Aerodinamicas/9(kCLsb)
  Gear Position/1 -> Fuerzas Aerodinamicas/17(Gear Position)
  Mux2/1 -> Scope7/1
  meters to feets/1 -> Terminator1/1
  meters to feets1/1 -> Scope/1
  meters to feets2/1 -> [Vz_ftmin], Scope4/1
  Angle Conversion7/1 -> [psi_deg]  "psi [deg]"
  [h] -> Saturation3/1
  [h] -> Fuerzas Aerodinamicas/5(Altura [m])
  Fuerzas Aerodinamicas/2(Dx) -> [D], Resistencia/1
  Giro de Fuerzas a Ejes Cuerpo QUATERNIONES/5(Mx_c) -> Subsystem3/2(Mx), Mx_c/1  "Mx"
  Giro de Fuerzas a Ejes Cuerpo QUATERNIONES/6(My_c) -> Subsystem13/2(My), My_c/1  "My"
  Giro de Fuerzas a Ejes Cuerpo QUATERNIONES/7(Mz_c) -> Subsystem4/2(Mz), Mz_c/1  "Mz"
  [Fx_c] -> Monitor de Fuerzas Ejes Cuerpo/1  "Fx"
  [Fy_c] -> Monitor de Fuerzas Ejes Cuerpo/2  "Fy"
  [Fz_c] -> Monitor de Fuerzas Ejes Cuerpo/3  "Fz"
  [Mx_c] -> Monitor de Fuerzas Ejes Cuerpo/4  "Mx"
  [My_c] -> Monitor de Fuerzas Ejes Cuerpo/5  "My"
  [Mz_c] -> Monitor de Fuerzas Ejes Cuerpo/6  "Mz"
  [Fx_c] -> Mux1/1
  [Fy_c] -> Mux1/2
  [Fz_c] -> Mux1/3
  [V_body] -> Quaternion Rotation1/2
  [Vx_global] -> Integrator2/1
  [Vy_global] -> Integrator1/1
  6DOF (Ejes Cuerpo)/7(p q r) -> [pqr]  "pqr [rad]"
  [pqr] -> Fuerzas Aerodinamicas/8(p q r)
  Fuerzas Aerodinamicas/6(Mz) -> Momento de Guiñada/1, [Mz]
  [Mz] -> Giro de Fuerzas a Ejes Cuerpo QUATERNIONES/6(Mz)
  [QuaterGiro_VC] -> Giro de Fuerzas a Ejes Cuerpo QUATERNIONES/10(Quaternion de Giro (Ejes Viento a Cuerpo))
  [QuaterGiro_GC] -> Giro de Fuerzas a Ejes Cuerpo QUATERNIONES/9(Quaternion de Giro (Ejes Globales a Cuerpo))
  [phi] -> Mux5/1
  [theta] -> Mux5/2
  [psi] -> Mux5/3
  Gain6/1 -> [Zpos]
  [Zpos] -> Mux4/3
  [Ypos] -> Mux4/2
  [Xpos] -> Mux4/1
  Mux5/1 -> Animacion Aeronave 3D Side/2, Animacion Aeronave 3D Back/2, Animacion Aeronave 3D ISO/2
  Mux4/1 -> Animacion Aeronave 3D Back/1, Animacion Aeronave 3D Side/1, Animacion Aeronave 3D ISO/1
  Nonlinear Second-Order Actuator1/1 -> [Rudder_Total], Fuerzas Aerodinamicas/15(Rudder Position)
  Nonlinear Second-Order Actuator2/1 -> [Aileron_Total], Fuerzas Aerodinamicas/16(Aileron Position)
  Saturation1/1 -> Nonlinear Second-Order Actuator1/1, Display6/1
  Saturation2/1 -> Nonlinear Second-Order Actuator2/1, Display7/1
  Elevator Position/1 -> Sum/2
  [Asist_Elev] -> Sum/1
  [alpha] -> Asistencia en Vuelo/1(alpha)  "alpha"
  Asistencia en Vuelo/1(Asis. Elevator) -> Mux6/1
  [Velocidad] -> Asistencia en Vuelo/3(V)  "V"
  [beta] -> Asistencia en Vuelo/2(beta)  "beta"
  Asistencia en Vuelo/2(Asis. Rudder) -> Mux6/2
  Rudder Position/1 -> Sum1/2
  Aileron Position/1 -> Sum2/2
  [psi_deg] -> Monitor General/3  "Psi"
  [phi_deg] -> Monitor General/1  "Phi"
  [theta_deg] -> Monitor General/2  "Theta"
  [beta] -> Monitor General/8  "Beta"
  [alpha] -> Monitor General/4  "Alpha"
  [Vz_global] -> Integrator3/1
  Asistencia en Vuelo/3(Asis. Aileron) -> Mux6/3
  Mux6/1 -> Control ON/OFF Asistencia en Vuelo/1
  Control ON/OFF Asistencia en Vuelo/1 -> Demux2/1
  Demux2/2 -> [Asist_Rud]
  Demux2/1 -> [Asist_Elev]
  Demux2/3 -> [Asist_Ail]
  Saturation3/1 -> meters to feets/1, Modelo Atmosfera ISA/3(h)
  From Multimedia File/1 -> Volumen Efecto 1/1
  [V] -> Fuerzas Aerodinamicas/3(V [m/s])
  [V] -> Gain7/1
  Gain7/1 -> Scope5/1
  Mux7/1 -> Scope8/1
  [phi_deg] -> Gain11/1
  [psi_deg] -> Gain10/1
  Gain10/1 -> Matriz de Cambio de Ejes Globales a Cuerpo QUATERNIONES/1(psi)
  Gain1/1 -> Matriz de Cambio de Ejes Globales a Cuerpo QUATERNIONES/2(theta)
  Gain11/1 -> Matriz de Cambio de Ejes Globales a Cuerpo QUATERNIONES/3(phi)
  Subsystem6/1(Wind Angles) -> Scope6/1, Gain15/1, Demux3/1
  Subsystem6/2(Velocity) -> Scope6/2, Display2/1, [Velocidad]
  Demux3/3 -> [chi_body]
  Demux3/2 -> [gamma_body]
  Demux3/1 -> [mu_body]
  [gamma_body] -> Gain12/1
  Gain12/1 -> Matriz de Cambio de Ejes Viento a Cuerpo QUATERNIONES/2(gamma)
  Gain13/1 -> Matriz de Cambio de Ejes Viento a Cuerpo QUATERNIONES/3(mu)
  [mu_body] -> Gain13/1
  [chi_body] -> Gain14/1
  Gain14/1 -> Matriz de Cambio de Ejes Viento a Cuerpo QUATERNIONES/1(xi)
  Gain15/1 -> Incidence Angles/1
  Subsystem6/3("Alpha, Beta") -> Display1/1, Demux4/1
  Demux4/1 -> [alpha]
  Demux4/2 -> [beta]
  [Aileron] -> Asistencia en Vuelo/5(Aileron)
  [Rudder] -> Asistencia en Vuelo/6(Rudder)
  [Asist_Rud] -> Sum1/1
  [Asist_Ail] -> Sum2/1
  [Zpos] -> Mux11/3
  [Ypos] -> Mux11/2
  Mux11/1 -> To Workspace/1
  [Xpos] -> Mux11/1
  Mux12/1 -> To Workspace1/1
  [Vx_global] -> Mux12/1
  [Vy_global] -> Mux12/2
  [Vz_global] -> Mux12/3
  Mux13/1 -> To Workspace2/1
  [Mx_global] -> Mux13/1
  [My_global] -> Mux13/2
  [Mz_global] -> Mux13/3
  Mux14/1 -> To Workspace3/1
  [theta_deg] -> Mux14/2
  Mux15/1 -> To Workspace4/1
  [psi_deg] -> Mux14/3
  [phi_deg] -> Mux14/1
  [chi_body] -> Mux15/3
  [gamma_body] -> Mux15/2
  [mu_body] -> Mux15/1
  Sum3/1 -> Sum2/3
  [Aileron_JoyStick] -> Sum3/1
  Constant/1 -> Sum3/2
  Constant1/1 -> Sum4/2
  [Rudder_JoyStick] -> Sum4/1
  Sum4/1 -> Sum1/3
  Constant2/1 -> Sum5/2
  Sum5/1 -> Sum/3
  [Elevator_JoyStick] -> Sum5/1
  [alpha] -> To Workspace5/1
  [beta] -> To Workspace6/1
  Constant4/1 -> Switch1/3
  Constant5/1 -> Switch2/3
  Fuerzas Aerodinamicas/1(Lz) -> [L], Sustentacion/1
  [Mz_c] -> Mux16/3
  [My_c] -> Mux16/2
  [Mx_c] -> Mux16/1
  Mux16/1 -> To Workspace7/1
  Saturation/1 -> Nonlinear Second-Order Actuator/1, Display5/1
  [beta] -> Mux7/2
  [My_c] -> Mux17/2
  [Mx_c] -> Mux17/1
  Mux17/1 -> Quaternion Rotation3/2
  Demux7/3 -> Monitor de Momentos Ejes Globales1/3, [Mz_global]  "Fz"
  [QuaterGiro_GC] -> Quaternion Inverse2/1
  Quaternion Inverse2/1 -> Quaternion Rotation3/1
  Quaternion Rotation3/1 -> Demux7/1
  Demux7/2 -> Monitor de Momentos Ejes Globales1/2, [My_global]  "Fy"
  Demux7/1 -> Monitor de Momentos Ejes Globales1/1, [Mx_global]  "Fx"
  "       "/1 -> Subsystem9/1(Initial Mass)
  "          "/1 -> Subsystem9/2(Fuel)
  "               "/1 -> Subsystem9/3(Cargo)
  Subsystem9/1(Real Mass) -> [mass]
  [mass] -> 6DOF (Ejes Cuerpo)/7(Mass)
  [Trac] -> Abs/1
  Subsystem9/2(Fuel Capacity) -> [fuel_capacity]
  [Engine_Porcent] -> "Engine %  "/1
  [fuel_capacity_perc] -> Fuel %/1
  [fuel_capacity] -> Fuel Alert/1(Fuel Capacity)
  Fuel Alert/1(Lamp Indicator) -> Scope13/1
  Engine Alert/1(Engine Indicator) -> Scope14/1
  [Engine_Porcent] -> Engine Alert/1(Engine)
  Subsystem11/1(Vz con Suelo) -> [Vz_global]
  [h] -> Subsystem3/1(Altura), Subsystem4/1(Altura), Subsystem13/1(Altura), Subsystem10/1(Altura)
  Subsystem10/1(Fz con Suelo) -> [Fz_c]  "Fz"
  [h] -> Subsystem11/2(Altura)
  [h] -> Subsystem12/1(Altura)
  Subsystem12/1(Vz con Suelo) -> Mux/3
  Subsystem13/1(My con Suelo) -> [My_c]  "My"
  [IAS] -> Fuel %1/1
  [fuel_capacity] -> Gain5/1
  Gain5/1 -> To Workspace8/1
  m/s to knots/1 -> Scope15/1
  Volumen Efecto 1/1 -> Product3/1
  Product3/1 -> Audio Device Writer/1
  [Engine_Porcent] -> Gain24/1
  Gain24/1 -> Product3/2
  [phi_deg] -> Asistencia en Vuelo/4(Phi)
  [Ypos] -> XY Navigation/2
  [Xpos] -> XY Navigation/1
  [Xpos] -> Normal1/1(x)
  [Ypos] -> Normal1/2(y)
  Normal1/1(|Acumulative Distance|) -> [XYpos]
  [h] -> Altitude Navigation/2
  [XYpos] -> Altitude Navigation/1
  [h] -> Fuel %2/1
  [h] -> Subsystem16/1(h [m])
  Subsystem16/1(Wind Direction [deg]) -> Wind Direction/1
  Gain25/1 -> Mux19/1, Wind Vectors/1, [WindVelocity_Global]
  Subsystem9/3(Fuel Flow [kg/s]) -> Fuel Flow/1
  [QuaterGiro_GC] -> Quaternion Rotation6/1
  Mux19/1 -> Quaternion Rotation6/2
  Constant6/1 -> Mux19/2
  Quaternion Rotation6/1 -> Wind Vectors1/1, [WindVelocity_Body]
  6DOF (Ejes Cuerpo)/1(Vx) -> Sum7/2  "Vx"
  Demux8/1 -> Sum7/1
  Demux8/2 -> Sum8/1
  Demux8/3 -> Sum9/1
  6DOF (Ejes Cuerpo)/3(Vz) -> Sum9/2  "Vz"
  [WindVelocity_Global] -> Demux9/1
  Sum10/1 -> [Vx_global]  "Vx"
  Demux9/1 -> Sum10/2
  Sum11/1 -> [Vy_global]  "Vx"
  Demux9/2 -> Sum11/2
  Subsystem16/2(Wind Vectors) -> Gain25/1
  [theta_deg] -> Gain1/1
  [h] -> Subsystem14/1(Altura)
  Angle Conversion6/1 -> Mux2/2, [theta_deg]  "theta [deg]"
  Subsystem14/1(theta con Suelo) -> [theta]
  [theta_deg] -> Subsystem13/3(theta)
  6DOF (Ejes Cuerpo)/2(Vy) -> Sum8/2  "Vy"
  [WindVelocity_Body] -> Demux8/1
  [V_body] -> Demux10/1
  Demux10/1 -> Monitor General/5  "Vx_b"
  Demux10/2 -> Monitor General/6  "Vy_b"
  Demux10/3 -> Monitor General/7  "Vz_b"
  [Xpos] -> Gain8/1
  Subsystem16/3("Latitude, Longitude [deg]") -> Wind Vectors2/1, [Lat_Lon_deg]
  [Lat_Lon_deg] -> To Workspace9/1
  Gain8/1 -> Subsystem16/2(X [m])
  [Ypos] -> Gain9/1
  Gain9/1 -> Subsystem16/3(Y [m])
  Angle Conversion1/1 -> Sum12/2  "psi [deg]"
  Sum12/1 -> Ejes Cuerpo/5  "psi [deg]"
  Constant7/1 -> Sum12/1
  Joystick Input/1 -> Subsystem2/1(Axes)
  Joystick Input/2 -> Subsystem2/2(Buttons)
  ? -> Subsystem2/3(POV)
  Subsystem2/2(Elevator) -> Display9/1, [Elevator_JoyStick]
  Subsystem2/3(Engine) -> Display8/1, [Engine_JoyStick]
  Subsystem2/4(Rudder) -> Display3/1, [Rudder_JoyStick]
  Subsystem2/5(Flaps) -> Display11/1, [Flaps_JoyStick]
  Saturation8/1 -> Display4/1, Transfer Fcn1/1
  Flaps Position/1 -> Sum13/1
  [Flaps_JoyStick] -> Sum13/2
  Sum13/1 -> Saturation8/1
  Subsystem3/1(Mx con Suelo) -> [Mx_c]  "Fz"
  Subsystem4/1(Mz con Suelo) -> [Mz_c]  "Fz"
  Product1/1 -> q/1
  Subsystem2/1(Aileron) -> Display10/1, [Aileron_JoyStick]
  Abs/1 -> Subsystem9/4(Engine)
  [theta_deg] -> Brake Force System/1(Theta)
  [QuaterGiro_GC] -> Brake Force System/2(Quaternion GC)
  [Fx_c] -> Brake Force System/3(Fx Body)
  [Fy_c] -> Brake Force System/4(Fy Body)
  [Fz_c_brake] -> Brake Force System/5(Fz Body)
  [h] -> Brake Force System/6(Altura)
  [IAS] -> Brake Force System/7(Velocidad IAS)
  [Mz_c] -> Mux17/3
  Mux1/1 -> Quaternion Rotation2/2
  Sum14/1 -> [Fx_c_Total], 6DOF (Ejes Cuerpo)/1(Fx Cuerpo)
  [Fx_c] -> Sum14/2
  [Fy_c] -> Sum15/2
  Sum15/1 -> [Fy_c_Total], 6DOF (Ejes Cuerpo)/2(Fy Cuerpo)
  [Fz_c] -> Sum16/2
  Sum16/1 -> [Fz_c_Total], 6DOF (Ejes Cuerpo)/3(Fz Cuerpo)
  Demux5/1 -> Sum14/1
  Demux5/2 -> Sum15/1
  Demux5/3 -> Sum16/1
  Subsystem2/6(Brakes) -> [Brakes_JoyStick], Display12/1
  [Brakes_JoyStick] -> [Brakes_Total], Product4/2
  Brake Force System/1(Body Brake Forces) -> Product4/1
  Product4/1 -> Display/1, Demux5/1
  [Vy_body] -> Brake Force System/8(Velocidad Vy Body)
  [h] -> Auto-Piloto/1(Altura [m])
  [Vz_ftmin] -> Auto-Piloto/3(Vz [ft/min])
  Auto-Piloto/1(ALT Elevator) -> Switch5/1, ALT/1
  Sum/1 -> Sum17/2
  Sum17/1 -> Saturation/1
  [Elevator_AutoPilot] -> Sum17/1
  Demux6/1 -> [Elevator_AutoPilot]
  Mux3/1 -> Switch8/1, Master/1
  [IAS] -> Auto-Piloto/2(Velocidad [m/s])
  Auto-Piloto/2(VEL Engine) -> Switch6/1, VEL/1
  Demux6/2 -> [Engine_AutoPilot]
  [psi_deg] -> Auto-Piloto/4(Psi [deg])
  Auto-Piloto/3(HDG Rudder) -> Switch7/1, HDG/1
  Demux6/3 -> [Rudder_AutoPilot]
  Sum2/1 -> Sum19/2
  Sum19/1 -> [Aileron], Saturation2/1
  From153/1 -> Sum19/1
  Sum1/1 -> Sum20/2
  Sum20/1 -> [Rudder], Saturation1/1
  [Rudder_AutoPilot] -> Sum20/1
  Temperature Conversion/1 -> Temperatura1/1
  [XYpos] -> To Workspace10/1
  Demux11/1 -> Auto-Piloto/5(Altura Autopiloto [ft])
  Demux11/2 -> Auto-Piloto/6(Velocidad Autopiloto [knots])
  Demux11/3 -> Auto-Piloto/7(Direccion Autopiloto [deg])
  Dirección Autopiloto/1 -> Mux8/3
  Velocidad Autopiloto/1 -> Mux8/2
  Altura Autopiloto/1 -> Mux8/1
  Switch4/1 -> Demux11/1
  Subsystem15/2(Mission ON/OFF) -> Auto-Piloto/8(Mission ON/OFF), Switch4/2
  [IAS] -> Subsystem15/1(IAS)
  [h] -> Subsystem15/2(h)
  Mux8/1 -> Switch4/3
  Subsystem15/1(Autopilot) -> Switch4/1
  ALT/1 -> Switch5/3
  Subsystem15/3(Autopilot ON/OF) -> Demux12/1
  VEL/1 -> Switch6/3
  Demux12/2 -> Switch5/2
  HDG/1 -> Switch7/3
  Demux12/3 -> Switch6/2
  Demux12/4 -> Switch7/2
  Switch6/1 -> Mux3/2
  Switch5/1 -> Mux3/1
  Switch7/1 -> Mux3/3
  Master/1 -> Switch8/3
  Demux12/1 -> Switch8/2
  Switch8/1 -> Demux6/1
  [XYpos] -> Subsystem15/3(Distance)
  Nonlinear Second-Order Actuator/1 -> [Elevator_Total], Fuerzas Aerodinamicas/14(Elevator Position)
  Subsystem17/2(Trac) -> Traccion/1, [Trac]
  [Mach] -> Subsystem17/1(Mach)
  [fuel_capacity] -> Subsystem17/2(Fuel Capacity)
  [h] -> Subsystem17/3(Altura)
  Constant3/1 -> Subsystem17/4(Engine Trim)
  Porcentaje de Motor/1 -> Subsystem17/6(Intrumet Panel Engine)
  [Engine_JoyStick] -> Subsystem17/7(Engine Joystick)
  Subsystem17/1(Fuel Capacity %) -> [fuel_capacity_perc]
  Subsystem17/3(Total Engine %) -> Engine %/1, [Engine_Porcent]
  [Engine_Porcent] -> Mux9/1
  [Elevator_Total] -> Mux9/2
  [Brakes_Total] -> Mux9/8
  [Speedbrake_Total] -> Mux9/7
  [Spoiler_Total] -> Mux9/6
  [Flaps_Total] -> Mux9/5
  [Rudder_Total] -> Mux9/4
  [Aileron_Total] -> Mux9/3
  Mux9/1 -> To Workspace12/1
  [Fx_c_Total] -> Mux10/1
  Mux10/1 -> To Workspace11/1
  [Fy_c_Total] -> Mux10/2
  [Fz_c_Total] -> Mux10/3
  [Engine_AutoPilot] -> Subsystem17/8(Engine Autopilot)
  [V_body] -> To Workspace13/1
  [theta_deg] -> Fuerzas Aerodinamicas/6(Alpha [deg])
  [beta] -> Fuerzas Aerodinamicas/7(Beta [deg])
  [Fz_global] -> Mux18/3
  [Fy_global] -> Mux18/2
  [Fx_global] -> Mux18/1
  Mux18/1 -> To Workspace14/1
